simulink model "smc_diff"  (R2024b)
settings: Solver=ode1  StartTime=0.0  StopTime=15  FixedStep=1e-5  RelTol=1e-3
libraries: simulink x1
settings Model: Creator=user  LastModifiedBy=user

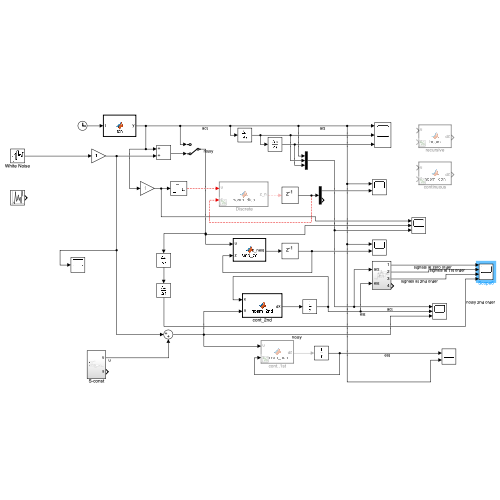
[thumbnail: Simulink's stored preview of the top-level diagram]
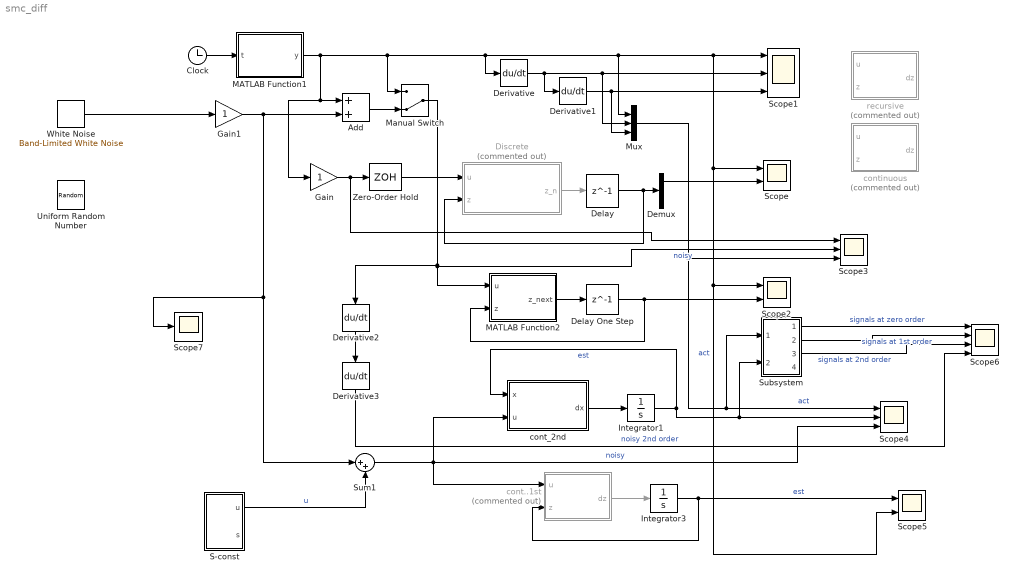
== system smc_diff ==
  " Discrete" : MATLAB Function  Commented=on  TreatAsAtomicUnit=on
  Add : Sum
  Clock : Clock
  Delay : Delay  DelayLength=1  InputProcessing=Columns as channels (frame based)
  Delay One Step : Delay  DelayLength=1
  Demux : Demux  Outputs=[1 2]
  Derivative{,1..3} (4 alike) : Derivative
  Gain : Gain
  Gain1 : Gain
  Integrator1 : Integrator
  Integrator3 : Integrator
  MATLAB Function1 : MATLAB Function  TreatAsAtomicUnit=on
  MATLAB Function2 : MATLAB Function  TreatAsAtomicUnit=on
  Manual Switch : ManualSwitch  CurrentSetting=0
  Mux : Mux  Inputs=3
  S-const : Subsystem
  Scope : Scope  NumInputPorts=2
  Scope1 : Scope  NumInputPorts=3
  Scope2 : Scope  NumInputPorts=2
  Scope3 : Scope  NumInputPorts=3
  Scope4 : Scope  NumInputPorts=3
  Scope5 : Scope  NumInputPorts=2
  Scope6 : Scope  NumInputPorts=4
  Scope7 : Scope
  Subsystem : Subsystem
  Sum1 : Sum  Inputs=|++
  Uniform Random Number : UniformRandomNumber  Minimum=-1e-3  Maximum=1e-3  SampleTime=0.001
  White Noise : simulink/Sources/Band-Limited White Noise  Cov=1e-8*1  Ts=0.001  seed=[23341]
  Zero-Order Hold : ZeroOrderHold  SampleTime=0.001
  cont..1st : MATLAB Function  Commented=on  TreatAsAtomicUnit=on
  cont_2nd : MATLAB Function  TreatAsAtomicUnit=on
  continuous : MATLAB Function  Commented=on  TreatAsAtomicUnit=on
  recursive : MATLAB Function  Commented=on  TreatAsAtomicUnit=on
  wires:
  " Discrete"/1(z_n) -> Delay/1
  Clock/1 -> MATLAB Function1/1(t)
  Delay/1 -> " Discrete"/2(z), Demux/1
  Derivative/1 -> Scope1/2, Mux/2, Derivative1/1
  Derivative1/1 -> Scope1/3, Mux/3
  Demux/1 -> Scope/2
  MATLAB Function2/1(z_next) -> Delay One Step/1
  Mux/1 -> Scope4/1, Subsystem/1(act), Scope3/3  "act"
  Delay One Step/1 -> Scope2/2, MATLAB Function2/2(z)
  cont_2nd/1(dx) -> Integrator1/1
  Integrator1/1 -> cont_2nd/1(x), Scope4/2, Subsystem/2(est)  "est"
  cont..1st/1(dz) -> Integrator3/1
  Integrator3/1 -> Scope5/1, cont..1st/2(z)  "est"
  Zero-Order Hold/1 -> " Discrete"/1(u)
  Sum1/1 -> cont..1st/1(u), Scope4/3, cont_2nd/2(u)  "noisy"
  Add/1 -> Manual Switch/2
  Gain/1 -> Zero-Order Hold/1, Scope3/1
  MATLAB Function1/1(y) -> Derivative/1, Mux/1, Scope/1, Scope2/1, Scope5/2, Scope1/1, Manual Switch/1, Gain/1, Add/1  "act"
  Manual Switch/1 -> Derivative2/1, MATLAB Function2/1(u), Scope3/2  "noisy"
  S-const/1(u) -> Sum1/2  "u"
  Subsystem/1(Out1) -> Scope6/1  "signals at zero order"
  Subsystem/2(Out2) -> Scope6/2  "signals at 1st order"
  Subsystem/3(Out3) -> Scope6/3  "signals at 2nd order"
  Derivative2/1 -> Derivative3/1
  Derivative3/1 -> Scope6/4  "noisy 2nd order"
  Gain1/1 -> Scope7/1, Sum1/1, Add/2
  White Noise/1 -> Gain1/1

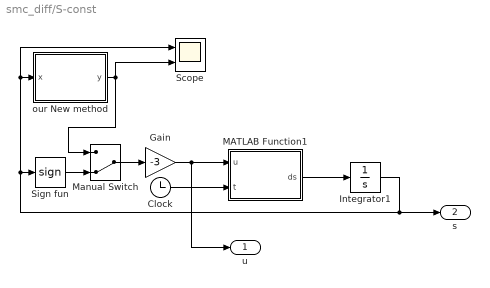
== system smc_diff/S-const ==
  Clock : Clock
  Gain : Gain  Gain=-3
  Integrator1 : Integrator  InitialCondition=5
  MATLAB Function1 : MATLAB Function  TreatAsAtomicUnit=on
  Manual Switch : ManualSwitch  CurrentSetting=0
  Scope : Scope  NumInputPorts=2
  Sign fun : Signum
  "our New method " : MATLAB Function  TreatAsAtomicUnit=on
  u : Outport
  s : Outport  Port=2
  wires:
  MATLAB Function1/1(ds) -> Integrator1/1
  Integrator1/1 -> Sign fun/1, Scope/1, "our New method "/1(x), s/1
  Clock/1 -> MATLAB Function1/2(t)
  Gain/1 -> MATLAB Function1/1(u), u/1
  "our New method "/1(y) -> Manual Switch/1, Scope/2
  Sign fun/1 -> Manual Switch/2
  Manual Switch/1 -> Gain/1

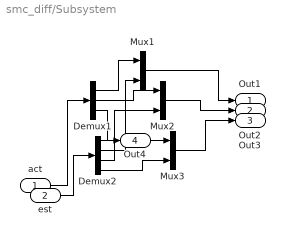
== system smc_diff/Subsystem ==
  act : Inport
  est : Inport  Port=2
  Demux1 : Demux  Outputs=3
  Demux2 : Demux  Outputs=[2 1 1 1]
  Mux1 : Mux  Inputs=2
  Mux2 : Mux  Inputs=2
  Mux3 : Mux  Inputs=2
  Out1 : Outport
  Out2 : Outport  Port=2
  Out3 : Outport  Port=3
  Out4 : Outport  Port=4
  wires:
  act/1 -> Demux1/1
  Demux1/2 -> Mux2/1
  Mux3/1 -> Out3/1
  Demux2/1 -> Out4/1
  Demux1/1 -> Mux1/1
  Demux2/4 -> Mux3/2
  Mux1/1 -> Out1/1
  Demux2/2 -> Mux1/2
  est/1 -> Demux2/1
  Mux2/1 -> Out2/1
  Demux1/3 -> Mux3/1
  Demux2/3 -> Mux2/2

== matlab function smc_diff/S-const/MATLAB Function1 ==
  data: u input; ds output; t input
function ds = fcn(u, t)
    %ds = cos(t) + (2 + sin(3*t))*u;
    ds = (1+exp(-2*t))*sin(2*t) + (5 + cos(t))*u;
end

== matlab function smc_diff/ Discrete ==
  data: u input; z_n output; z input
function z_n  = hosm_disc(u, z)
% Zero-Order Discrete Sliding Mode Differentiator Implementation

gamma = 1;  % Stability parameter
tau = 1e-5;   % Sampling time
L = 30;       % Gain parameter

% Ensure z is properly initialized
z_n = zeros(3, 1);  % Initialize as a column vector

% Compute next states using the given discrete update laws
% z(1) = z_2; % z(2) = z_1; % z(3) = z_0
z_n(1) = z(1) + (exp(-gamma * tau) * z(1) + (1/gamma) * (1 - exp(-gamma * tau)) * u) * tau;

z_n(2) = z(2) + (-1.5 * L^(1/2) * (abs(z(2) - z(1)))^(1/2)*sign(z(2) - z(1)) - gamma * z(1) + z(3)) * tau;

z_n(3) = z(3) - 1.1 * L * sign(z(2) - z(1)) * tau;


end

== matlab function smc_diff/MATLAB Function1 ==
  data: t input; y output
function y = fcn(t)

%y = -cos(t)/(2+sin(3*t));
y = -(1+exp(-2*t))*sin(2*t)/(5+cos(t));

== matlab function smc_diff/MATLAB Function2 ==
  data: u input; z_next output; z input
function z_next = smd_zo(u, z)
% Zero-Order Discrete Sliding Mode Estimator using Equation (22)
% u     - Input signal (f)
% z     - Previous estimated value of f (z0)
% tau   - Sampling time
% alpha - Tuning parameter

% Tuning parameters
alpha = 160; % Adjust for stability
tau = 1e-5;   % Sampling time
%L = 30;       % Gain parameter


% Compute next state using Equation (22)
z_next = exp(-alpha * tau) * z + (1 - exp(-alpha * tau)) * u;

end

== matlab function smc_diff/continuous ==
  data: u input; dz output; z input
function dz = hosm_con(u, z)
    % Extract system order
    L = 1;
    lambda = [1.1 3.06, 4.16 3];
    k = length(lambda) - 1;  
    
    % Initialize derivative vector
    dz = zeros(5, 1);
    
    error = z(2) - z(1);  % z0 - f(t)
    
    % Compute the differential equations
    % for i = 0:k-1
    %     exponent = (k-i) / (k+1);
    %     exponent1 = (i+1) / (k+1);
    %     dz(i+1) = -lambda(k+1-i) * L^exponent1 * (abs(error)^exponent * sign(error)) + z(i+2);
    % end
    gamma = 1;
    dz(1) = u - gamma*z(1);
    dz(2) = -lambda(4) * L^1/4 * (abs(error)^3/4 * sign(error)) + z(3)-gamma*z(1);
    dz(3) = -lambda(3) * L^2/4 * (abs(error)^2/4 * sign(error)) + z(4);
    dz(4) = -lambda(2) * L^3/4 * (abs(error)^1/4 * sign(error)) + z(5);
    % Last equation
    dz(5) = -lambda(1) * L * sign(error); 
end

== matlab function smc_diff/S-const/our New method  ==
  data: x input; y output
% function y = bisigmoid(x)
%     k = 1e4; c = 1;
%     y = tanh(k * x);
% end

function y = alevantbook(x)

  y = x/(abs(x)+1e-8);

end

== matlab function smc_diff/cont_2nd ==
  data: x input; u input; dx output
function dx = hosm_2nd(x, u)
% equivControlObserver implements Equation (14) for k=3.
%
% INPUTS:
%   t      - time (not used explicitly, but required for the Simulink function)
%   x      - state vector, a 5x1 vector:
%            x(1) = z_minus2 (auxiliary variable)
%            x(2) = z_minus1 (first state of differentiator)
%            x(3) = z_0      (second state, estimate of u_eq)
%            x(4) = z_1      (third state, estimate of u_eq derivative)
%            x(5) = z_2      (fourth state, estimate of u_eq second derivative)
%   u      - input control signal u(t) (scalar)
%   gamma  - positive scalar parameter (mostly, 1)
%   L      - known positive constant (bound on derivative)
%   lambda - vector of parameters [lambda0, lambda1, lambda2, lambda3]
%            corresponding to the differentiator gains.
%
dx = zeros(5, 1);
% OUTPUT:
%   dx     - derivative of state vector (5x1)
L = 35;
gamma = 1;
lambda = [1.1 3.06, 4.16 3];
k = length(lambda) - 1;  
% Extract states for clarity:
z_m2 = x(1);   % z_{-2}
z_m1 = x(2);   % z_{-1}
z0   = x(3);   % z_0, estimate of u_eq
z1   = x(4);   % z_1, estimate of u_eq derivative
z2   = x(5);   % z_2, estimate of u_eq second derivative

% Extract lambda parameters:
lambda0 = lambda(1);
lambda1 = lambda(2);
lambda2 = lambda(3);
lambda3 = lambda(4);

% Compute the error term for the differentiator.
% Here the error is defined as e = z_m1 - z_m2.
e = z_m1 - z_m2;

% Define the fractional power function:
% fpower(w, alpha) = |w|^alpha * sign(w)
fpower = @(w, alpha) (abs(w)^alpha) * sign(w);

%-----------------------------------------------------------------------
% Equation for z_{-2} (auxiliary filter):
dz_m2 = u - gamma * z_m2;

%-----------------------------------------------------------------------
% Differentiator dynamics (modified version of eq (6) with input replaced by z_{-2})
% Note: The additional term - gamma*z_m2 is added only to the first differentiator
% equation (corresponding to the e0 component).
%
% The following equations implement:
%
%   dot{z}_{-1} = -lambda3*L^(1/4)*fpower(e, 3/4) + z0 - gamma*z_m2,
%   dot{z}_0    = -lambda2*L^(2/4)*fpower(e, 2/4) + z1,
%   dot{z}_1    = -lambda1*L^(3/4)*fpower(e, 1/4) + z2,
%   dot{z}_2    = -lambda0*L*sign(e).
%
dz_m1 = -lambda3 * L^(1/4) * fpower(e, 3/4) + z0 - gamma * z_m2;
dz0   = -lambda2 * L^(2/4) * fpower(e, 2/4) + z1;
dz1   = -lambda1 * L^(3/4) * fpower(e, 1/4) + z2;
dz2   = -lambda0 * L * sign(e);

%-----------------------------------------------------------------------
% Assemble the state derivative vector:
dx = [dz_m2; dz_m1; dz0; dz1; dz2];

end

== matlab function smc_diff/recursive ==
  data: u input; dz output; z input
function dz = hosm(u, z)
    % Extract system order
    L = 30;
    lambda = [1.1 1.5 2 3];
    k = length(lambda) - 1;  
    
    % Initialize derivative vector
    dz = zeros(6, 1);
    
    error = z(2) - dz(1);  % z0 - f(t)
    error2 = z(3) - dz(2);
    error3 = z(4) - dz(3);
    error4 = z(5) - dz(4);
    
    % Compute the differential equations
    % for i = 0:k-1
    %     exponent = (k-i) / (k+1-i);
    %     exponent1 = (1) / (k+1-i);
    %     dz(i+1) = -lambda(k+1-i) * L^exponent1 * (abs(error)^exponent * sign(error)) + z(i+2);
    % end
    gamma = 1;
    dz(1) = u - gamma*z(1);
    dz(2) = -lambda(4) * L^1/4 * (abs(error)^3/4 * sign(error)) + z(3)-gamma*z(1);
    dz(3) = -lambda(3) * L^1/3 * (abs(error2)^2/3 * sign(error2)) + z(4);
    dz(4) = -lambda(2) * L^1/2 * (abs(error3)^1/2 * sign(error3)) + z(5);
    % Last equation
    dz(5) = -lambda(1) * L * sign(error4);
end

== matlab function smc_diff/cont..1st ==
  data: u input; dz output; z input
function dz = hosm_con(u, z)
    % Extract system order
    L = 30;
    lambda = [1.1 1.5];
    k = length(lambda) - 1;  
    
    % Initialize derivative vector
    dz = zeros(3, 1);
    
    error = z(2) - z(1);  % z0 - f(t)
    
    % Compute the differential equations
    % for i = 0:k-1
    %     exponent = (k-i) / (k+1);
    %     exponent1 = (i+1) / (k+1);
    %     dz(i+1) = -lambda(k+1-i) * L^exponent1 * (abs(error)^exponent * sign(error)) + z(i+2);
    % end
    gamma = 1;
    dz(1) = u - gamma*z(1);
    dz(2) = -lambda(2) * L^1/2 * abs(error)^1/2 * sign(error) + z(3)-gamma*z(1);
    dz(3) = -lambda(1) * L * sign(error);
end
